simulink model "DLQR_disturbance_rejection_simulink"  (R2023b)
settings: Solver=FixedStepAuto  StartTime=0.0  StopTime=60  FixedStep=1/1000  RelTol=1e-3
values from neighbouring files (symbols this model uses):
  h = 0.125    [Controllers_Design.m]    (also in DLMI_code_validation.m = 1; DLQR_rotational_controller_design.m = Pc_inv(end,:); DLQR_translational_controller.m = Pc_inv(end,:))
  m = 1220.24/1000    (= 1.22024)    [Controllers_Design.m]    (also in calculate_inclination_force.m; forceCompensationDueGlassInclination.m)
  tractor_max_force = 0.2238    [Controllers_Design.m]
  ts = 0.0521    [Controllers_Design.m]
undefined symbols (not defined in the file or in its folder): Gm, K_trans, tm
libraries: simulink_extras x2
settings Model: Creator=luanv  LastModifiedBy=luanv

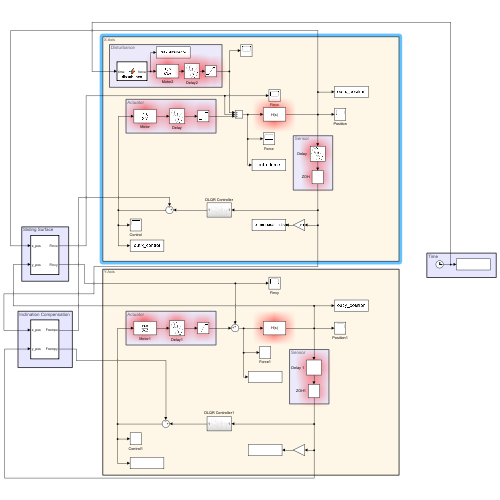
[thumbnail: Simulink's stored preview of the top-level diagram]
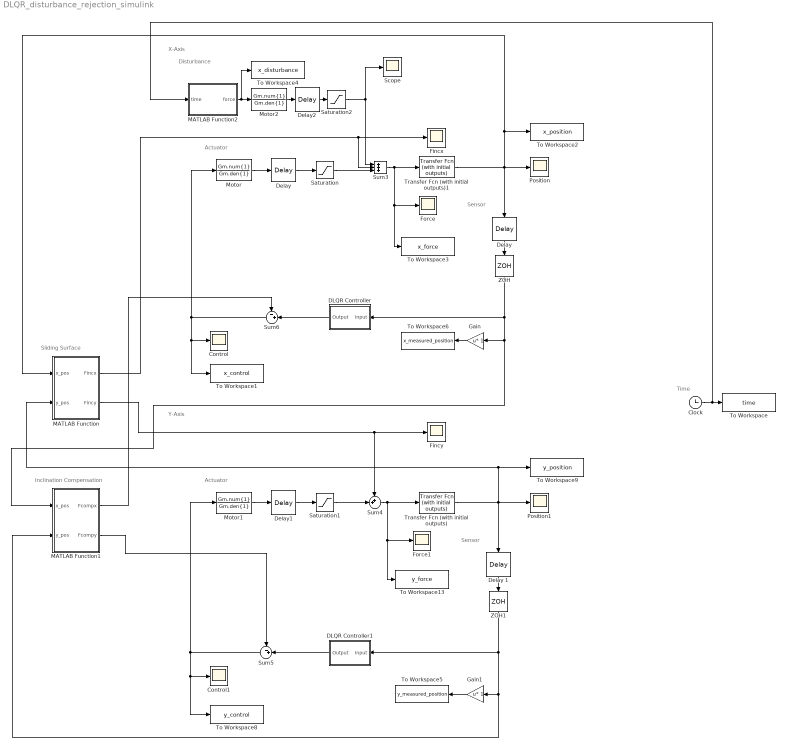
== system DLQR_disturbance_rejection_simulink ==
  note: Disturbance
  note: Actuator
  note: Y-Axis
  note: X-Axis
  note: Actuator
  note: Sensor
  note: Inclination Compensation
  note: Sensor
  note: Sliding Surface
  note: Time
  Clock : Clock
  Control : Scope
  Control1 : Scope
  DLQR Controller : Subsystem
  DLQR Controller1 : Subsystem
  Delay : TransportDelay  DelayTime=tm
  "Delay " : TransportDelay  DelayTime=ts
  Delay 1 : TransportDelay  DelayTime=ts
  Delay1 : TransportDelay  DelayTime=tm
  Delay2 : TransportDelay  DelayTime=tm
  Fincx : Scope
  Fincy : Scope
  Force : Scope
  Force1 : Scope
  Gain : Gain  Multiplication=Matrix(u*K)
  Gain1 : Gain  Multiplication=Matrix(u*K)
  MATLAB Function : MATLAB Function  TreatAsAtomicUnit=on
  MATLAB Function1 : MATLAB Function  TreatAsAtomicUnit=on
  MATLAB Function2 : MATLAB Function  TreatAsAtomicUnit=on
  Motor : TransferFcn  Numerator=Gm.num{1}  Denominator=Gm.den{1}
  Motor1 : TransferFcn  Numerator=Gm.num{1}  Denominator=Gm.den{1}
  Motor2 : TransferFcn  Numerator=Gm.num{1}  Denominator=Gm.den{1}
  Position : Scope
  Position1 : Scope
  Saturation : Saturate  UpperLimit=tractor_max_force  LowerLimit=-tractor_max_force
  Saturation1 : Saturate  UpperLimit=tractor_max_force  LowerLimit=-tractor_max_force
  Saturation2 : Saturate  UpperLimit=tractor_max_force  LowerLimit=-tractor_max_force
  Scope : Scope
  Sum3 : Sum  Inputs=+++
  Sum4 : Sum  Inputs=++|
  Sum5 : Sum  Inputs=-+|
  Sum6 : Sum  Inputs=-+|
  To Workspace : ToWorkspace  VariableName=time  SaveFormat=Timeseries  SampleTime=-1
  To Workspace1 : ToWorkspace  VariableName=x_control  SaveFormat=Timeseries  SampleTime=1/1000
  To Workspace13 : ToWorkspace  VariableName=y_force  SaveFormat=Timeseries  SampleTime=-1
  To Workspace2 : ToWorkspace  VariableName=x_position  SaveFormat=Timeseries  SampleTime=-1
  To Workspace3 : ToWorkspace  VariableName=x_force  SaveFormat=Timeseries  SampleTime=-1
  To Workspace4 : ToWorkspace  VariableName=x_disturbance  SaveFormat=Timeseries  SampleTime=1/1000
  To Workspace5 : ToWorkspace  VariableName=y_measured_position  SaveFormat=Timeseries  SampleTime=1/1000
  To Workspace6 : ToWorkspace  VariableName=x_measured_position  SaveFormat=Timeseries  SampleTime=1/1000
  To Workspace8 : ToWorkspace  VariableName=y_control  SaveFormat=Timeseries  SampleTime=1/1000
  To Workspace9 : ToWorkspace  VariableName=y_position  SaveFormat=Timeseries  SampleTime=-1
  Transfer Fcn (with initial outputs) : simulink_extras/Additional Linear/Transfer Fcn (with initial outputs)  N=[1]  D=[m 0 0]  Y0=0  U0=0
  Transfer Fcn (with initial outputs)1 : simulink_extras/Additional Linear/Transfer Fcn (with initial outputs)  N=[1]  D=[m 0 0]  Y0=0  U0=0
  ZOH : ZeroOrderHold  SampleTime=h
  ZOH1 : ZeroOrderHold  SampleTime=h
  wires:
  MATLAB Function/1(Fincx) -> Fincx/1, Sum3/2
  Delay 1/1 -> ZOH1/1
  Sum6/1 -> Motor/1, To Workspace1/1, Control/1
  MATLAB Function1/1(Fcompx) -> Sum6/1
  Sum3/1 -> To Workspace3/1, Force/1, Transfer Fcn (with initial outputs)1/1
  Motor1/1 -> Delay1/1
  MATLAB Function/2(Fincy) -> Sum4/1, Fincy/1
  MATLAB Function1/2(Fcompy) -> Sum5/1
  Sum4/1 -> To Workspace13/1, Force1/1, Transfer Fcn (with initial outputs)/1
  Sum5/1 -> Motor1/1, Control1/1, To Workspace8/1
  Saturation/1 -> Sum3/3
  "Delay "/1 -> ZOH/1
  DLQR Controller/1(Output) -> Sum6/2
  Delay/1 -> Saturation/1
  Clock/1 -> MATLAB Function2/1(time), To Workspace/1
  Saturation1/1 -> Sum4/2
  Delay1/1 -> Saturation1/1
  Motor/1 -> Delay/1
  Transfer Fcn (with initial outputs)/1 -> To Workspace9/1, MATLAB Function/2(y_pos), Position1/1, Delay 1/1
  Transfer Fcn (with initial outputs)1/1 -> MATLAB Function/1(x_pos), To Workspace2/1, "Delay "/1, Position/1
  DLQR Controller1/1(Output) -> Sum5/2
  ZOH/1 -> DLQR Controller/1(Input), Gain/1, MATLAB Function1/1(x_pos)
  Motor2/1 -> Delay2/1
  Delay2/1 -> Saturation2/1
  Saturation2/1 -> Sum3/1, Scope/1
  Gain/1 -> To Workspace6/1
  Gain1/1 -> To Workspace5/1
  ZOH1/1 -> DLQR Controller1/1(Input), Gain1/1, MATLAB Function1/2(y_pos)
  MATLAB Function2/1(force) -> To Workspace4/1, Motor2/1

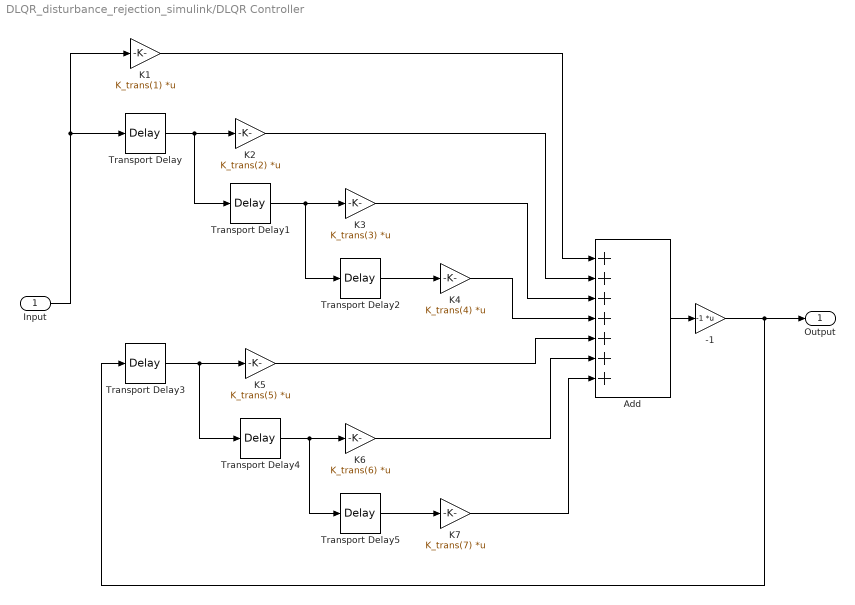
== system DLQR_disturbance_rejection_simulink/DLQR Controller ==
  Input : Inport
  -1 : Gain  Gain=-1  Multiplication=Matrix(K*u)
  Add : Sum  Inputs=+++++++
  K1 : Gain  Gain=K_trans(1)  Multiplication=Matrix(K*u)
  K2 : Gain  Gain=K_trans(2)  Multiplication=Matrix(K*u)
  K3 : Gain  Gain=K_trans(3)  Multiplication=Matrix(K*u)
  K4 : Gain  Gain=K_trans(4)  Multiplication=Matrix(K*u)
  K5 : Gain  Gain=K_trans(5)  Multiplication=Matrix(K*u)
  K6 : Gain  Gain=K_trans(6)  Multiplication=Matrix(K*u)
  K7 : Gain  Gain=K_trans(7)  Multiplication=Matrix(K*u)
  Transport Delay{,1..5} (6 alike) : TransportDelay  DelayTime=h
  Output : Outport
  wires:
  Input/1 -> Transport Delay/1, K1/1
  Transport Delay/1 -> Transport Delay1/1, K2/1
  Transport Delay1/1 -> Transport Delay2/1, K3/1
  Transport Delay2/1 -> K4/1
  Transport Delay3/1 -> Transport Delay4/1, K5/1
  Transport Delay4/1 -> Transport Delay5/1, K6/1
  Transport Delay5/1 -> K7/1
  K1/1 -> Add/1
  K2/1 -> Add/2
  K3/1 -> Add/3
  K4/1 -> Add/4
  K5/1 -> Add/5
  K6/1 -> Add/6
  K7/1 -> Add/7
  Add/1 -> -1/1
  -1/1 -> Transport Delay3/1, Output/1

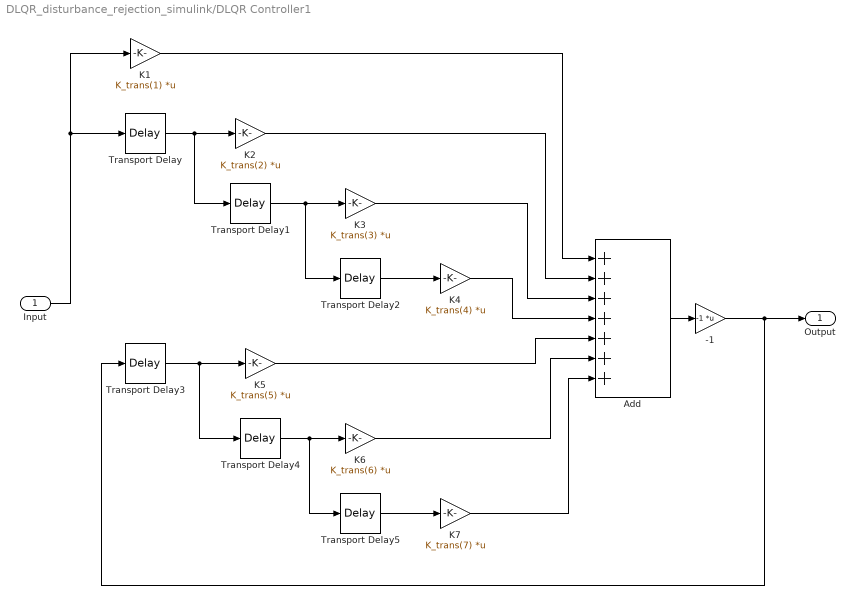
== system DLQR_disturbance_rejection_simulink/DLQR Controller1 ==
  Input : Inport
  -1 : Gain  Gain=-1  Multiplication=Matrix(K*u)
  Add : Sum  Inputs=+++++++
  K1 : Gain  Gain=K_trans(1)  Multiplication=Matrix(K*u)
  K2 : Gain  Gain=K_trans(2)  Multiplication=Matrix(K*u)
  K3 : Gain  Gain=K_trans(3)  Multiplication=Matrix(K*u)
  K4 : Gain  Gain=K_trans(4)  Multiplication=Matrix(K*u)
  K5 : Gain  Gain=K_trans(5)  Multiplication=Matrix(K*u)
  K6 : Gain  Gain=K_trans(6)  Multiplication=Matrix(K*u)
  K7 : Gain  Gain=K_trans(7)  Multiplication=Matrix(K*u)
  Transport Delay{,1..5} (6 alike) : TransportDelay  DelayTime=h
  Output : Outport
  wires:
  Input/1 -> Transport Delay/1, K1/1
  Transport Delay/1 -> Transport Delay1/1, K2/1
  Transport Delay1/1 -> Transport Delay2/1, K3/1
  Transport Delay2/1 -> K4/1
  Transport Delay3/1 -> Transport Delay4/1, K5/1
  Transport Delay4/1 -> Transport Delay5/1, K6/1
  Transport Delay5/1 -> K7/1
  K1/1 -> Add/1
  K2/1 -> Add/2
  K3/1 -> Add/3
  K4/1 -> Add/4
  K5/1 -> Add/5
  K6/1 -> Add/6
  K7/1 -> Add/7
  Add/1 -> -1/1
  -1/1 -> Transport Delay3/1, Output/1

== matlab function DLQR_disturbance_rejection_simulink/MATLAB Function1 ==
  data: x_pos input; y_pos input; Fcompx output; Fcompy output
function [Fcompx,Fcompy] = compensation(x_pos,y_pos)

    coder.extrinsic('forceCompensationDueGlassInclination')
    
    Fcompx = 0;
    Fcompy = 0;
    
    [Fcompx,Fcompy] = forceCompensationDueGlassInclination(x_pos,y_pos);

end

== matlab function DLQR_disturbance_rejection_simulink/MATLAB Function ==
  data: x_pos input; y_pos input; Fincx output; Fincy output
function [Fincx,Fincy] = inclination(x_pos,y_pos)

    coder.extrinsic('calculate_inclination_force')
    
    Fincx = 0;
    Fincy = 0;
    
    [Fincx,Fincy] = calculate_inclination_force(x_pos,y_pos);

end

== matlab function DLQR_disturbance_rejection_simulink/MATLAB Function2 ==
  data: time input; force output
function force  = disturbance(time)

    maxForce = 2 * 0.1255; 
	frequency = 0.2732;
    force = 0;
	amplitude = 2*(maxForce/16);

	if ((time >= 0) && (time < 6))
        force = 0;
    end

	if ((time >= 6.0) && (time < (6.0 + (4 * pi) / frequency)))	
		force = amplitude * sin(frequency * time - 6.0 * frequency);
    end

	if (time >= (6.0 + (4 * pi) / frequency))
		force = 0;
    end   

end
